simulink model "Zalacznik_10"  (R2022a)
settings: Solver=ode5  StartTime=0.0  StopTime=20  FixedStep=0.001  RelTol=1e-3  EnableMultiTasking=on
undefined symbols (not defined in the file or in its folder): Kd, Ki, Kp
settings Model: Creator=Michal  LastModifiedBy=Michal
settings SolverCC: AlgebraicLoopSolver=TrustRegion
settings DataIOCC: LimitDataPoints=on  SaveFormat=Array  SignalLoggingSaveFormat=ModelDataLogs  ReturnWorkspaceOutputs=off
settings OptimizationCC: ExpressionDepthLimit=2147483647  LifeSpan=inf
settings DebuggingCC: UnderspecifiedInitializationDetection=Classic  MergeDetectMultiDrivingBlocksExec=none  SolverPrmCheckMsg=warning  FcnCallInpInsideContextMsg=warning  UnconnectedInputMsg=warning  UnconnectedOutputMsg=warning  UnconnectedLineMsg=warning  StateNameClashWarn=warning  SFUnexpectedBacktrackingDiag=warning  SFNoUnconditionalDefaultTransitionDiag=warning  SFExecutionAtInitializationDiag=none  SFMachineParentedDataDiag=warning  ArithmeticOperatorsInVariantConditions=warning
settings HardwareCC: ProdBitPerPointer=32  ProdBitPerSizeT=32  ProdBitPerPtrDiffT=32  ProdLargestAtomicFloat=None  ProdIntDivRoundTo=Undefined  ProdEndianess=Unspecified  ProdWordSize=32  ProdHWDeviceType=32-bit Generic
settings ModelReferenceCC: PropagateSignalLabelsOutOfModel=off
settings SFSimCC: SimUseLocalCustomCode=off  CustomCodeUndefinedFunction=UseInterfaceOnly
settings RTWCC: RTWUseLocalCustomCode=off
settings CodeAppCC: StateflowObjectComments=on
settings GRTTargetCC: TargetLangStandard=C89/C90 (ANSI)  CombineOutputUpdateFcns=off  GRTInterface=on
settings ConfigComp: CovMetricSettings=dw  CovSaveCumulativeToWorkspaceVar=on  CovSaveSingleToWorkspaceVar=on  CovExternalEMLEnable=off

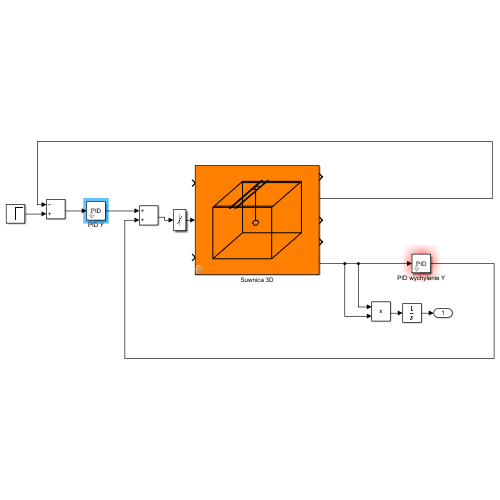
[thumbnail: Simulink's stored preview of the top-level diagram]
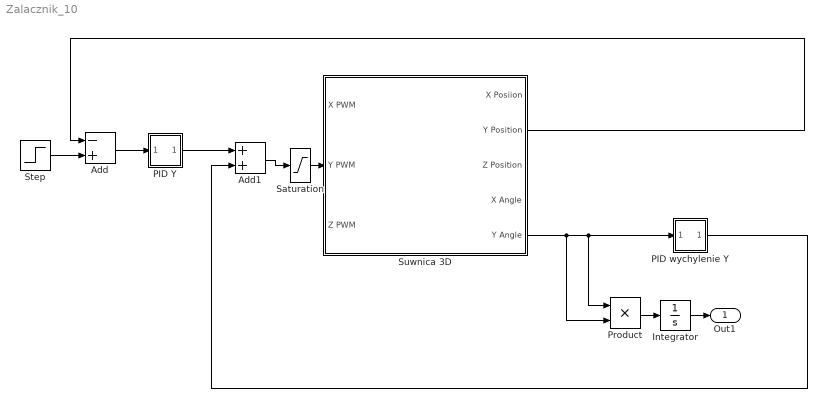
== system Zalacznik_10 ==
  Add : Sum  Inputs=-+
  Add1 : Sum
  Integrator : Integrator
  PID Y : Subsystem  mask(PID Controller){P=24.005, I=23.676, D=0.452}
      mask prompts: P "Proportional:"; I "Integral:"; D "Derivative:"
      mask help:
      | Enter expressions for proportional, integral, and derivative terms.
      | P+I/s+Ds
      mask Help: This block implements a PID controller where parameters are entered for the Proportional, Integral and Derivative terms. Unmask this block to see how it works. The derivative term is implemented using a true derivative block.
      mask Display: disp('PID')
  PID wychylenie Y : Subsystem  mask(PID Controller){P=Kp, I=Ki, D=Kd}
      mask prompts: P "Proportional:"; I "Integral:"; D "Derivative:"
      mask help:
      | Enter expressions for proportional, integral, and derivative terms.
      | P+I/s+Ds
      mask Help: This block implements a PID controller where parameters are entered for the Proportional, Integral and Derivative terms. Unmask this block to see how it works. The derivative term is implemented using a true derivative block.
      mask Display: disp('PID')
  Product : Product
  Saturation : Saturate  UpperLimit=1  LowerLimit=-1
  Step : Step  After=0.4  SampleTime=0
  Suwnica 3D : Subsystem  mask{RR=off, x0=[0.1, 0.1, 0.01,  0.1, 0.1, 0.1, 0.1, 0.1,  0.1, 0.1, -1]}
      mask prompts: RR "Model with constant length"; x0 "Initial conditions:[x,x',y,y',alfa,alfa',beta,beta',z,z',t]"
      mask Display: plot( [0 1], [0 0], [0 1], [1 1], [0 0], [0 1], [1 1], [0 1], [0.5 1.5], [0.5 0.5], [0.5 1.5], [1.5 1.5], [0.5 0.5], [0.5 1.5], [1.5 1.5], [0.5 1.5], [0 0.5], [0 0.5], [1 1.5], [0 0.5], [0 0.5], [1 1.5], [1 1.5], [1 1.5], [0.02 1.02], [1.02 1.02], [0.48 1.48], [1.48 1.48], [0.27 0.83], [0.97 1.53], [0.29 0.85], [0.97 1.53], [0.37 0.93], [0.97 1.53], [0.39 0.95], [0.97 1.53], [0.65 0.75], [1.35 1.35], [0.7 0.8], [1.4 1.4], [0.725 0.725], [1.375 0.75], 0.725+0.05*sin([0:0.5:7]), 0.7+0.05*cos([0:0.5:7]), [-0.3 -0.3], [-0.3 -0.3], [1.8 1.8], [1.8 1.8] )
  Out1 : Outport
  wires:
  Step/1 -> Add/2
  Saturation/1 -> Suwnica 3D/2(Y PWM)
  Suwnica 3D/2(Y Position) -> Add/1
  Integrator/1 -> Out1/1
  Product/1 -> Integrator/1
  Add/1 -> PID Y/1(In_1)
  Suwnica 3D/5(Y Angle) -> Product/2, Product/1, PID wychylenie Y/1(In_1)
  Add1/1 -> Saturation/1
  PID Y/1(Out_1) -> Add1/1
  PID wychylenie Y/1(Out_1) -> Add1/2

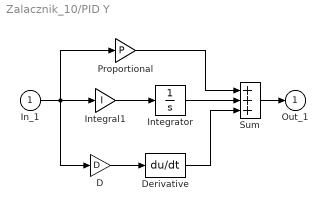
== system Zalacznik_10/PID Y ==
  In_1 : Inport
  D : Gain  Gain=D  SaturateOnIntegerOverflow=on  OutDataTypeStr=Inherit: Same as input  ParamDataTypeStr=Inherit: Same as input
  Derivative : Derivative
  Integral1 : Gain  Gain=I  SaturateOnIntegerOverflow=on  OutDataTypeStr=Inherit: Same as input  ParamDataTypeStr=Inherit: Same as input
  Integrator : Integrator  LimitOutput=on  UpperSaturationLimit=0.3  LowerSaturationLimit=-0.3
  Proportional : Gain  Gain=P  SaturateOnIntegerOverflow=on  OutDataTypeStr=Inherit: Same as input  ParamDataTypeStr=Inherit: Same as input
  Sum : Sum  Inputs=+++  InputSameDT=on  SaturateOnIntegerOverflow=on  OutDataTypeStr=Inherit: Same as first input
  Out_1 : Outport  InitialOutput=0
  wires:
  Proportional/1 -> Sum/1
  Integrator/1 -> Sum/2
  Derivative/1 -> Sum/3
  In_1/1 -> Proportional/1, Integral1/1, D/1
  Sum/1 -> Out_1/1
  D/1 -> Derivative/1
  Integral1/1 -> Integrator/1

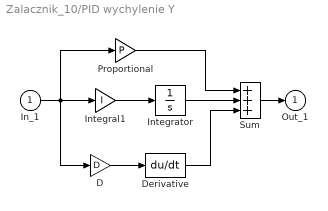
== system Zalacznik_10/PID wychylenie Y ==
  In_1 : Inport
  D : Gain  Gain=D  SaturateOnIntegerOverflow=on  OutDataTypeStr=Inherit: Same as input  ParamDataTypeStr=Inherit: Same as input
  Derivative : Derivative
  Integral1 : Gain  Gain=I  SaturateOnIntegerOverflow=on  OutDataTypeStr=Inherit: Same as input  ParamDataTypeStr=Inherit: Same as input
  Integrator : Integrator  LimitOutput=on  UpperSaturationLimit=0.3  LowerSaturationLimit=-0.3
  Proportional : Gain  Gain=P  SaturateOnIntegerOverflow=on  OutDataTypeStr=Inherit: Same as input  ParamDataTypeStr=Inherit: Same as input
  Sum : Sum  Inputs=+++  InputSameDT=on  SaturateOnIntegerOverflow=on  OutDataTypeStr=Inherit: Same as first input
  Out_1 : Outport  InitialOutput=0
  wires:
  Proportional/1 -> Sum/1
  Integrator/1 -> Sum/2
  Derivative/1 -> Sum/3
  In_1/1 -> Proportional/1, Integral1/1, D/1
  Sum/1 -> Out_1/1
  D/1 -> Derivative/1
  Integral1/1 -> Integrator/1

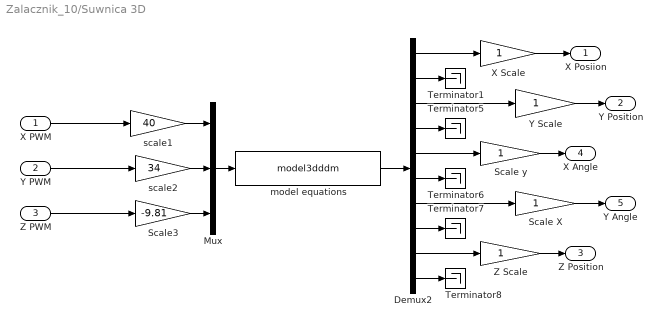
== system Zalacznik_10/Suwnica 3D ==
  X PWM : Inport
  Y PWM : Inport  Port=2
  Z PWM : Inport  Port=3
  Demux2 : Demux  Outputs=10
      settings: DisplayOption=none
  Mux : Mux  Inputs=3
  Scale X : Gain  SaturateOnIntegerOverflow=on  OutDataTypeStr=Inherit: Same as input  ParamDataTypeStr=Inherit: Same as input
  Scale y : Gain  SaturateOnIntegerOverflow=on  OutDataTypeStr=Inherit: Same as input  ParamDataTypeStr=Inherit: Same as input
  Scale3 : Gain  Gain=-9.81  SaturateOnIntegerOverflow=on  OutDataTypeStr=Inherit: Same as input  ParamDataTypeStr=Inherit: Same as input
  Terminator{1,5..8} (5 alike) : Terminator
  X Scale : Gain  SaturateOnIntegerOverflow=on  OutDataTypeStr=Inherit: Same as input  ParamDataTypeStr=Inherit: Same as input
  Y Scale : Gain  SaturateOnIntegerOverflow=on  OutDataTypeStr=Inherit: Same as input  ParamDataTypeStr=Inherit: Same as input
  Z Scale : Gain  SaturateOnIntegerOverflow=on  OutDataTypeStr=Inherit: Same as input  ParamDataTypeStr=Inherit: Same as input
  model equations : S-Function  FunctionName=model3dddm  Parameters=x0(1) x0(2) x0(3) x0(4) x0(5) x0(6) x0(7) x0(8) x0(9) x0(10) x0(11) RR  SFunctionDeploymentMode=off  EnableBusSupport=off
  scale1 : Gain  Gain=40  SaturateOnIntegerOverflow=on  OutDataTypeStr=Inherit: Same as input  ParamDataTypeStr=Inherit: Same as input
  scale2 : Gain  Gain=34  SaturateOnIntegerOverflow=on  OutDataTypeStr=Inherit: Same as input  ParamDataTypeStr=Inherit: Same as input
  X Posiion : Outport  Tag=X Position
  Y Position : Outport  Port=2
  Z Position : Outport  Port=3
  X Angle : Outport  Port=4
  Y Angle : Outport  Port=5
  wires:
  Mux/1 -> model equations/1
  Y Scale/1 -> Y Position/1
  model equations/1 -> Demux2/1
  X Scale/1 -> X Posiion/1
  Demux2/1 -> X Scale/1
  Demux2/3 -> Y Scale/1
  Z Scale/1 -> Z Position/1
  Demux2/9 -> Z Scale/1
  Scale y/1 -> X Angle/1
  Demux2/5 -> Scale y/1
  Scale X/1 -> Y Angle/1
  Demux2/7 -> Scale X/1
  Demux2/2 -> Terminator1/1
  Demux2/4 -> Terminator5/1
  Demux2/6 -> Terminator6/1
  Demux2/8 -> Terminator7/1
  Demux2/10 -> Terminator8/1
  scale2/1 -> Mux/2
  Y PWM/1 -> scale2/1
  Scale3/1 -> Mux/3
  Z PWM/1 -> Scale3/1
  scale1/1 -> Mux/1
  X PWM/1 -> scale1/1
